simulink library "Theoretical_Collector_Optics"  (Simulink 8.2)
settings: Solver=ode45  StartTime=0.0  StopTime=10.0  RelTol=1e-3
libraries: carnot x1
settings Model: Creator=lena.frank  LastModifiedBy=drhf

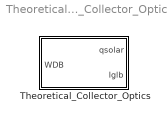
== system Theoretical_Collector_Optics ==
  Theoretical_Collector_Optics : Subsystem  mask(theoretical collector optics){FTA=0.8, ncover=1, refin=1.525, d=0.004, ext=4}
      mask prompts: FTA "Fin Efficiency * Transmission * Absorption (FTA) [-]"; ncover "Number of covers [-]"; refin "Refraction index of material [-]"; d "Thickness of the material in m"; ext "Extinction coefficient in 1/m"
      mask help:
      | Transforms direct and diffuse radiation to an absorbed solar power per unit area. FTA or F'(TauAlfa) is defined from the incidence angle modifiers Kdir and Kdfu:
      | FTA = eta0 / (Kdir(15°)*0.85 + Kdfu*0.15)
      | Kdir (for direct radiation) and Kdfu (for diffuse radiation) are derived from Fresnels equations refraction index (glass = 1.526), the thickness and the extinction coefficient (extra white glass 4/m, float glass 16/m).
      | See "taualfa" in the manual or type "help taualfa" on the command line for more information on the calculation of the IAM.
      mask init:
      | teta = [0:5:90]; % incidence angle
      | KL = d*ext; % extiction * thickness
      | kb = taualfa (ncover, refin, teta*pi/180, KL, 1);
      | kd = taualfa (ncover, refin, pi/3, KL, 1);
      | kd = kd/kb(1);
      | kb = kb/kb(1);
      mask Help: web(fullfile(path_carnot('help'),'Theoretical_Collector_Optics.html'),'-helpbrowser')

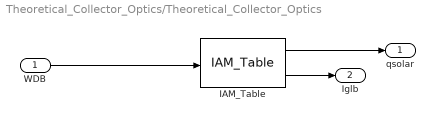
== system Theoretical_Collector_Optics/Theoretical_Collector_Optics ==
  WDB : Inport
  IAM_Table : carnot/Source/Solar_Thermal/IncidenceAngleModifier/IAM_Table  fta=FTA  angle=teta  Kb=kb  Kd=kd
  qsolar : Outport
  Iglb : Outport  Port=2
  wires:
  IAM_Table/2 -> Iglb/1
  IAM_Table/1 -> qsolar/1
  WDB/1 -> IAM_Table/1
